simulink model "SimAllanVariance"  (Simulink 8.8)
settings: Solver=VariableStepAuto  StartTime=0.0  StopTime=Tf  RelTol=1e-3
values from neighbouring files (symbols this model uses):
  Fs = 10    [AllanVariance.m]    (also in simulador.m = 250)
  Ts = 1/Fs    (= 0.1)    [AllanVariance.m]    (also in AllanVarianceDemo.m = [sqrt(3);1;NaN;3;sqrt(2)]; procesamientoDatos.m = 0.01; simulador.m = 0.004)
  TSim = TSimHs*3600    (= 1800)    [AllanVariance.m]    (also in simulador.m = 5; simuladorRuido.m = TSim*3600)
libraries: dspsrcs4 x5, simulink x1
settings Model: SuppressorTable=22 serialization::archive 11 0 3 0 0 0 11 0  Creator=root  LastModifiedBy=root
settings DataIOCC: LimitDataPoints=off  SaveFormat=Dataset  SignalLoggingSaveFormat=Dataset
settings OptimizationCC: LifeSpan=auto
settings DebuggingCC: UnderspecifiedInitializationDetection=Simplified  MergeDetectMultiDrivingBlocksExec=error  FcnCallInpInsideContextMsg=error  StateNameClashWarn=none  SFUnexpectedBacktrackingDiag=error  SFNoUnconditionalDefaultTransitionDiag=error  SFExecutionAtInitializationDiag=warning
settings HardwareCC: ProdBitPerPointer=64  ProdBitPerSizeT=64  ProdBitPerPtrDiffT=64  ProdLargestAtomicFloat=Float  ProdIntDivRoundTo=Zero  ProdEndianess=LittleEndian  ProdWordSize=64  ProdHWDeviceType=Intel->x86-64 (Windows64)
settings ModelReferenceCC: PropagateSignalLabelsOutOfModel=on
settings GRTTargetCC: TargetLangStandard=C99 (ISO)  GeneratePreprocessorConditionals=Use local settings  CombineOutputUpdateFcns=on  GRTInterface=off
settings ConfigComp: CovMetricSettings=dwe  CovHtmlReporting=off  CovSaveCumulativeToWorkspaceVar=off  CovSaveSingleToWorkspaceVar=off  CovExternalEMLEnable=on

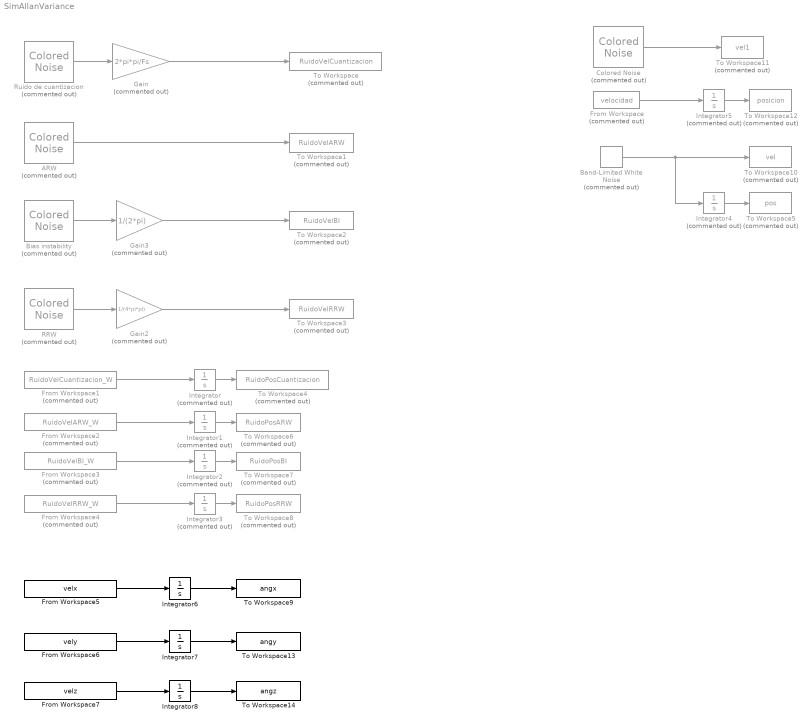
== system SimAllanVariance ==
  ARW : dspsrcs4/Colored Noise  Commented=on  Color=custom  InverseFrequencyPower=0  NumChannels=1  OutputDataType=double  SamplesPerFrame=TSim/Ts  SampleTime=Ts  RandomStream=mt19937ar with seed  Seed=80  SimulateUsing=Interpreted execution
  Band-Limited White Noise : simulink/Sources/Band-Limited White Noise  Commented=on  Cov=[0.1]  Ts=0.1  seed=[23341]
  Bias instability : dspsrcs4/Colored Noise  Commented=on  Color=custom  InverseFrequencyPower=1  NumChannels=1  OutputDataType=double  SamplesPerFrame=TSim/Ts  SampleTime=Ts  RandomStream=mt19937ar with seed  Seed=70  SimulateUsing=Interpreted execution
  Colored Noise : dspsrcs4/Colored Noise  Commented=on  Color=custom  InverseFrequencyPower=1  NumChannels=1  OutputDataType=double  SamplesPerFrame=TSim/Ts  SampleTime=Ts  RandomStream=mt19937ar with seed  Seed=67  SimulateUsing=Interpreted execution
  From Workspace : FromWorkspace  Commented=on  VariableName=velocidad
  From Workspace1 : FromWorkspace  Commented=on  VariableName=RuidoVelCuantizacion_W
  From Workspace2 : FromWorkspace  Commented=on  VariableName=RuidoVelARW_W
  From Workspace3 : FromWorkspace  Commented=on  VariableName=RuidoVelBI_W
  From Workspace4 : FromWorkspace  Commented=on  VariableName=RuidoVelRRW_W
  From Workspace5 : FromWorkspace  VariableName=velx  OutDataTypeStr=double  SampleTime=.1
  From Workspace6 : FromWorkspace  VariableName=vely  OutDataTypeStr=double  SampleTime=.1
  From Workspace7 : FromWorkspace  VariableName=velz  OutDataTypeStr=double  SampleTime=.1
  Gain : Gain  Commented=on  Gain=2*pi*pi/Fs
  Gain2 : Gain  Commented=on  Gain=1/(4*pi*pi)
  Gain3 : Gain  Commented=on  Gain=1/(2*pi)
  Integrator{,1..5} (6 alike) : Integrator  Commented=on
  Integrator6 : Integrator
  Integrator7 : Integrator
  Integrator8 : Integrator
  RRW : dspsrcs4/Colored Noise  Commented=on  Color=custom  InverseFrequencyPower=2  NumChannels=1  OutputDataType=double  SamplesPerFrame=TSim/Ts  SampleTime=Ts  RandomStream=mt19937ar with seed  Seed=60  SimulateUsing=Interpreted execution
  Ruido de cuantizacion : dspsrcs4/Colored Noise  Commented=on  Color=custom  InverseFrequencyPower=-2  NumChannels=1  OutputDataType=double  SamplesPerFrame=TSim/Ts  SampleTime=Ts  RandomStream=mt19937ar with seed  Seed=67  SimulateUsing=Interpreted execution
  To Workspace : ToWorkspace  Commented=on  VariableName=RuidoVelCuantizacion  SaveFormat=Timeseries  SampleTime=Ts
      settings: Save2DSignal=2-D array (concatenate along first dimension)
  To Workspace1 : ToWorkspace  Commented=on  VariableName=RuidoVelARW  SaveFormat=Timeseries  SampleTime=Ts
      settings: Save2DSignal=2-D array (concatenate along first dimension)
  To Workspace10 : ToWorkspace  Commented=on  VariableName=vel  SampleTime=Ts
      settings: MaxDataPoints=TSim/Ts  Save2DSignal=2-D array (concatenate along first dimension)
  To Workspace11 : ToWorkspace  Commented=on  VariableName=vel1  SampleTime=Ts
      settings: MaxDataPoints=TSim/Ts  Save2DSignal=2-D array (concatenate along first dimension)
  To Workspace12 : ToWorkspace  Commented=on  VariableName=posicion  SampleTime=Ts
      settings: MaxDataPoints=TSim/Ts  Save2DSignal=2-D array (concatenate along first dimension)
  To Workspace13 : ToWorkspace  VariableName=angy  SampleTime=.1
      settings: Save2DSignal=2-D array (concatenate along first dimension)
  To Workspace14 : ToWorkspace  VariableName=angz  SampleTime=.1
      settings: Save2DSignal=2-D array (concatenate along first dimension)
  To Workspace2 : ToWorkspace  Commented=on  VariableName=RuidoVelBI  SaveFormat=Timeseries  SampleTime=Ts
      settings: Save2DSignal=2-D array (concatenate along first dimension)
  To Workspace3 : ToWorkspace  Commented=on  VariableName=RuidoVelRRW  SaveFormat=Timeseries  SampleTime=Ts
      settings: Save2DSignal=2-D array (concatenate along first dimension)
  To Workspace4 : ToWorkspace  Commented=on  VariableName=RuidoPosCuantizacion  SampleTime=Ts
      settings: Save2DSignal=2-D array (concatenate along first dimension)
  To Workspace5 : ToWorkspace  Commented=on  VariableName=pos  SampleTime=Ts
      settings: MaxDataPoints=TSim/Ts  Save2DSignal=2-D array (concatenate along first dimension)
  To Workspace6 : ToWorkspace  Commented=on  VariableName=RuidoPosARW  SampleTime=Ts
      settings: Save2DSignal=2-D array (concatenate along first dimension)
  To Workspace7 : ToWorkspace  Commented=on  VariableName=RuidoPosBI  SampleTime=Ts
  To Workspace8 : ToWorkspace  Commented=on  VariableName=RuidoPosRRW  SampleTime=Ts
  To Workspace9 : ToWorkspace  VariableName=angx  SampleTime=.1
      settings: Save2DSignal=2-D array (concatenate along first dimension)
  wires:
  ARW/1 -> To Workspace1/1
  Bias instability/1 -> Gain3/1
  RRW/1 -> Gain2/1
  Gain2/1 -> To Workspace3/1
  Gain3/1 -> To Workspace2/1
  Ruido de cuantizacion/1 -> Gain/1
  Gain/1 -> To Workspace/1
  Integrator4/1 -> To Workspace5/1
  Band-Limited White Noise/1 -> Integrator4/1, To Workspace10/1
  Colored Noise/1 -> To Workspace11/1
  From Workspace/1 -> Integrator5/1
  Integrator5/1 -> To Workspace12/1
  Integrator3/1 -> To Workspace8/1
  From Workspace1/1 -> Integrator/1
  From Workspace4/1 -> Integrator3/1
  From Workspace3/1 -> Integrator2/1
  From Workspace2/1 -> Integrator1/1
  Integrator2/1 -> To Workspace7/1
  Integrator1/1 -> To Workspace6/1
  Integrator/1 -> To Workspace4/1
  From Workspace5/1 -> Integrator6/1
  Integrator6/1 -> To Workspace9/1
  From Workspace6/1 -> Integrator7/1
  Integrator7/1 -> To Workspace13/1
  From Workspace7/1 -> Integrator8/1
  Integrator8/1 -> To Workspace14/1
